simulink model "Project1_week3_sim"  (R2023b)
settings: Solver=VariableStepAuto  StartTime=0.0  StopTime=25  RelTol=1e-3
values from neighbouring files (symbols this model uses):
  A = [0.0, 100,0,100]    [P1_week3_code.m]
  b = [10,0.1]    [P1_week3_code.m]
  bool = 1    [P1_week3_code.m]
  freq = [0.1,100]    [P1_week3_code.m]
  J = [100,0.01]    [P1_week3_code.m]
  w_0 = [10.0,0.0]    [P1_week3_code.m]
settings Model: Creator=rahma  LastModifiedBy=rahma

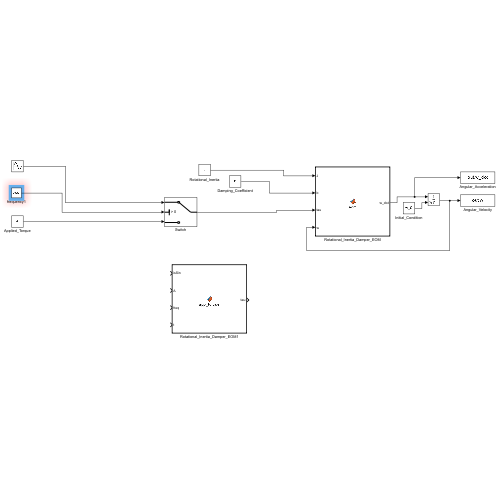
[thumbnail: Simulink's stored preview of the top-level diagram]
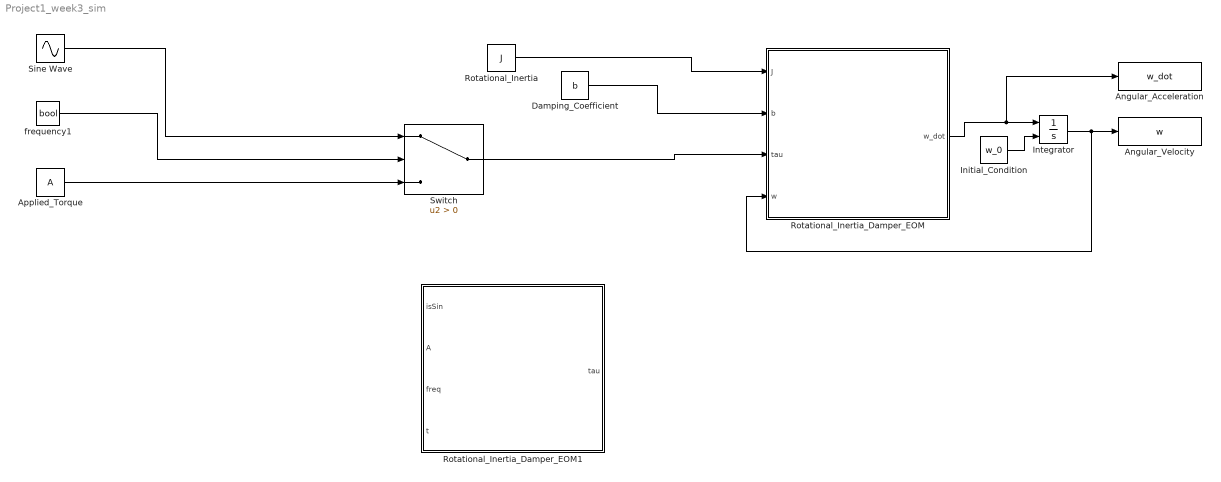
== system Project1_week3_sim ==
  Angular_Acceleration : ToWorkspace  VariableName=w_dot  SaveFormat=Timeseries  SampleTime=-1
  Angular_Velocity : ToWorkspace  VariableName=w  SaveFormat=Timeseries  SampleTime=-1
  Applied_Torque : Constant  Value=A
  Damping_Coefficient : Constant  Value=b
  Initial_Condition : Constant  Value=w_0
  Integrator : Integrator  InitialConditionSource=external
  Rotational_Inertia : Constant  Value=J
  Rotational_Inertia_Damper_EOM : MATLAB Function  TreatAsAtomicUnit=on
  Rotational_Inertia_Damper_EOM1 : MATLAB Function  TreatAsAtomicUnit=on
  Sine Wave : Sin  Amplitude=A  Frequency=freq  SampleTime=0
  Switch : Switch  Criteria=u2 > Threshold  SaturateOnIntegerOverflow=off  InputSameDT=off
  frequency1 : Constant  Value=bool
  wires:
  Initial_Condition/1 -> Integrator/2
  Rotational_Inertia_Damper_EOM/1(w_dot) -> Angular_Acceleration/1, Integrator/1
  Damping_Coefficient/1 -> Rotational_Inertia_Damper_EOM/2(b)
  Applied_Torque/1 -> Switch/3
  Rotational_Inertia/1 -> Rotational_Inertia_Damper_EOM/1(J)
  Integrator/1 -> Rotational_Inertia_Damper_EOM/4(w), Angular_Velocity/1
  Sine Wave/1 -> Switch/1
  frequency1/1 -> Switch/2
  Switch/1 -> Rotational_Inertia_Damper_EOM/3(tau)

== matlab function Project1_week3_sim/Rotational_Inertia_Damper_EOM1 ==
  data: isSin input; A input; freq input; tau output; t input
function tau = app_torque(isSin, A, freq, t)
if isSin == 0
    tau = A;
else 
    tau = A*sin(freq*t);
end

== matlab function Project1_week3_sim/Rotational_Inertia_Damper_EOM ==
  data: J input; w_dot output; b input; tau input; w input
function w_dot = eom(J, b, tau, w)
% Recall EOM: J*w_dot = tau_applied - tau_damped
tau_damped = b.*w;
% tau = A.*sin(freq.*t);
w_dot = (1/J)*(tau - tau_damped);
end
